simulink model "spindle"  (Simulink 7.6)
settings: Solver=ode14x  StartTime=0.0  StopTime=10  FixedStep=1.0/1024  RelTol=1e-3
libraries: simulink x2, dsparch4 x1
settings Model: Creator=admin  LastModifiedBy=minos001
settings SolverCC: ExtrapolationOrder=1
settings DebuggingCC: StrictBusMsg=Warning

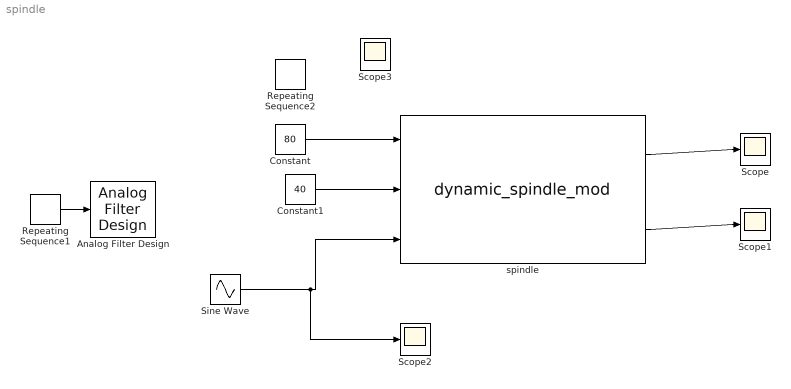
== system spindle ==
  Analog Filter Design : dsparch4/Analog Filter Design  method=Butterworth  filttype=Lowpass  N=3  Wlo=2*pi*15  Whi=80  Rp=2  Rs=40
  Constant : Constant  Value=80
  Constant1 : Constant  Value=40
  Repeating Sequence1 : simulink/Sources/Repeating Sequence  SystemSampleTime=-1  rep_seq_t=[0.0, 0.1, 0.4, 0.5, 1.0]  rep_seq_y=[1.0, 1.1, 1.1, 1.0, 1.0]
  Repeating Sequence2 : simulink/Sources/Repeating Sequence  SystemSampleTime=-1  rep_seq_t=[0 1 1.01 2]  rep_seq_y=[80 80 40 40]
  Scope{,1..3} (4 alike) : Scope
      Scope settings: TimeRange=2  SaveName=fr_Ia  MaxDataPoints=4000
      Scope1 settings: TimeRange=3  SaveName=fr_II  MaxDataPoints=4000
      Scope2 settings: TimeRange=10  SaveName=muscle_length  MaxDataPoints=4000
      Scope3 settings: TimeRange=3  SaveName=ScopeData3
  Sine Wave : Sin  Amplitude=0.1  Bias=1.1  Frequency=2*pi*2  SampleTime=0
  spindle : S-Function  FunctionName=dynamic_spindle_mod  Parameters=[10.4649 10.4649 10.4649] [0.1127 0.1623 0.1623] [0.0605 0.0822 0.0822] [0.2356 -0.046 -0.069] [0 0 0] [0.0289 0.0636 0.0954] [1 0.7 0.7] [1 0.92 0.92] [20000 10000 10000] [20000 7250 7250] [0.3 0.3 0.3] [0.46 0.46 0.46] [0.04 0.04 0.04] [0.76 0.76 0.76] [1 0.04 0.04] [0.192 0.185 0.0001] [0.0002 0.0002 0.0002] [1 0.5 1] [1]  EnableBusSupport=off
      mask Display:
      | port_label('input', 1, 'gamma dynamic');
      | port_label('input', 2, 'gamma static');
      | port_label('input', 3, 'Lce(L0)');
      | port_label('output',1,'Ia');
      | port_label('output',2,'II');
      | disp('Muscle Spindle \n(S-Function)')
  wires:
  Constant/1 -> spindle/1
  spindle/1 -> Scope/1
  spindle/2 -> Scope1/1
  Repeating Sequence1/1 -> Analog Filter Design/1
  Constant1/1 -> spindle/2
  Sine Wave/1 -> spindle/3, Scope2/1
